simulink model "generic_truck_src"  (Simulink 10.3)
settings: Solver=ode45  StartTime=0.0  StopTime=inf  RelTol=1e-3  EnableMultiTasking=on
libraries: TruckMaker4SL x1, simulink x1
(part 2 of 2)

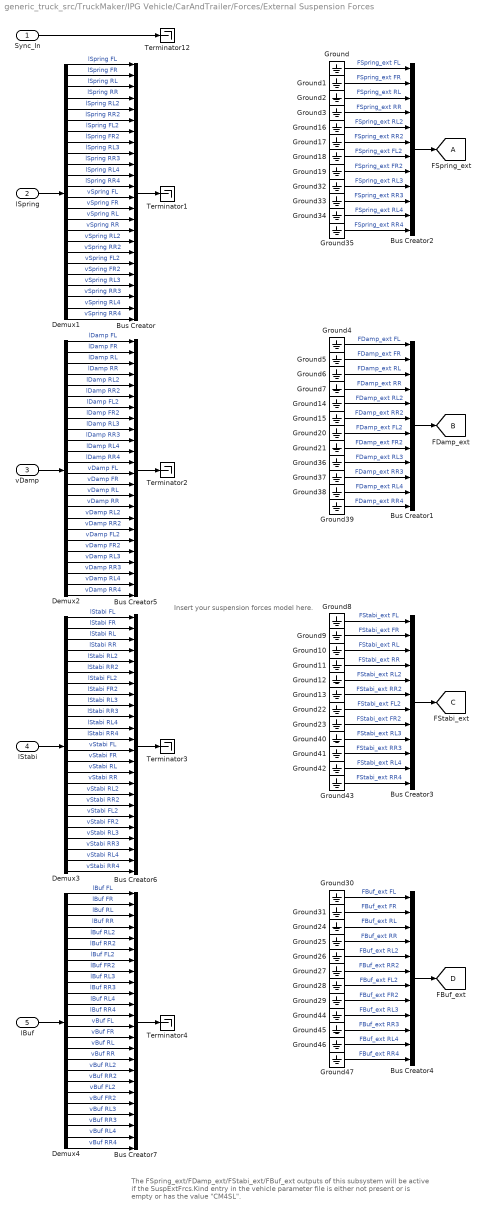
== system generic_truck_src/TruckMaker/IPG Vehicle/CarAndTrailer/Forces/External Suspension Forces ==
  note: The FSpring_ext/FDamp_ext/FStabi_ext/FBuf_ext outputs of this subsystem will be
      | active if the SuspExtFrcs.Kind entry in the vehicle parameter file
      | is either not present or is empty or has the value "CM4SL".
  note: Insert your suspension forces model here.
  Sync_In : Inport
  lSpring : Inport  Port=2
  vDamp : Inport  Port=3
  lStabi : Inport  Port=4
  lBuf : Inport  Port=5
  Bus Creator{,5..7} (4 alike) : BusCreator  Inputs=24
  Bus Creator{1..4} (4 alike) : BusCreator  Inputs=12
  Demux{1..4} (4 alike) : Demux  Outputs=24
      settings: DisplayOption=none
  Ground{,1..47} (48 alike) : Ground
  Terminator{1..4,12} (5 alike) : Terminator
  tag scope: A=global, B=global, C=global, D=global
  wires:
  Ground46/1 -> Bus Creator4/11  "FBuf_ext RL4"
  Ground47/1 -> Bus Creator4/12  "FBuf_ext RR4"
  Ground45/1 -> Bus Creator4/10  "FBuf_ext RR3"
  Ground44/1 -> Bus Creator4/9  "FBuf_ext RL3"
  Ground42/1 -> Bus Creator3/11  "FStabi_ext RL4"
  Ground43/1 -> Bus Creator3/12  "FStabi_ext RR4"
  Ground41/1 -> Bus Creator3/10  "FStabi_ext RR3"
  Ground40/1 -> Bus Creator3/9  "FStabi_ext RL3"
  Ground38/1 -> Bus Creator1/11  "FDamp_ext RL4"
  Ground39/1 -> Bus Creator1/12  "FDamp_ext RR4"
  Ground37/1 -> Bus Creator1/10  "FDamp_ext RR3"
  Ground36/1 -> Bus Creator1/9  "FDamp_ext RL3"
  Ground35/1 -> Bus Creator2/12  "FSpring_ext RR4"
  Ground34/1 -> Bus Creator2/11  "FSpring_ext RL4"
  Ground33/1 -> Bus Creator2/10  "FSpring_ext RR3"
  Ground32/1 -> Bus Creator2/9  "FSpring_ext RL3"
  Demux4/24 -> Bus Creator7/24  "vBuf RR4"
  Demux4/23 -> Bus Creator7/23  "vBuf RL4"
  Demux4/22 -> Bus Creator7/22  "vBuf RR3"
  Demux4/21 -> Bus Creator7/21  "vBuf RL3"
  Demux4/20 -> Bus Creator7/20  "vBuf FR2"
  Demux4/19 -> Bus Creator7/19  "vBuf FL2"
  Demux4/18 -> Bus Creator7/18  "vBuf RR2"
  Demux4/17 -> Bus Creator7/17  "vBuf RL2"
  Demux3/24 -> Bus Creator6/24  "vStabi RR4"
  Demux3/23 -> Bus Creator6/23  "vStabi RL4"
  Demux3/22 -> Bus Creator6/22  "vStabi RR3"
  Demux3/21 -> Bus Creator6/21  "vStabi RL3"
  Demux3/20 -> Bus Creator6/20  "vStabi FR2"
  Demux3/19 -> Bus Creator6/19  "vStabi FL2"
  Demux3/18 -> Bus Creator6/18  "vStabi RR2"
  Demux3/17 -> Bus Creator6/17  "vStabi RL2"
  Demux2/24 -> Bus Creator5/24  "vDamp RR4"
  Demux2/23 -> Bus Creator5/23  "vDamp RL4"
  Demux2/22 -> Bus Creator5/22  "vDamp RR3"
  Demux2/21 -> Bus Creator5/21  "vDamp RL3"
  Demux2/20 -> Bus Creator5/20  "vDamp FR2"
  Demux2/19 -> Bus Creator5/19  "vDamp FL2"
  Demux2/18 -> Bus Creator5/18  "vDamp RR2"
  Demux2/17 -> Bus Creator5/17  "vDamp RL2"
  Demux1/24 -> Bus Creator/24  "vSpring RR4"
  Demux1/23 -> Bus Creator/23  "vSpring RL4"
  Demux1/22 -> Bus Creator/22  "vSpring RR3"
  Demux1/21 -> Bus Creator/21  "vSpring RL3"
  Demux1/20 -> Bus Creator/20  "vSpring FR2"
  Demux1/19 -> Bus Creator/19  "vSpring FL2"
  Demux1/18 -> Bus Creator/18  "vSpring RR2"
  Demux1/17 -> Bus Creator/17  "vSpring RL2"
  Demux3/10 -> Bus Creator6/10  "lStabi RR3"
  Demux4/16 -> Bus Creator7/16  "vBuf RR"
  Demux4/15 -> Bus Creator7/15  "vBuf RL"
  Demux4/14 -> Bus Creator7/14  "vBuf FR"
  Demux4/13 -> Bus Creator7/13  "vBuf FL"
  Demux4/12 -> Bus Creator7/12  "lBuf RR4"
  Demux4/11 -> Bus Creator7/11  "lBuf RL4"
  Demux4/10 -> Bus Creator7/10  "lBuf RR3"
  Demux4/9 -> Bus Creator7/9  "lBuf RL3"
  Demux3/16 -> Bus Creator6/16  "vStabi RR"
  Demux3/15 -> Bus Creator6/15  "vStabi RL"
  Demux3/14 -> Bus Creator6/14  "vStabi FR"
  Demux3/13 -> Bus Creator6/13  "vStabi FL"
  Demux3/12 -> Bus Creator6/12  "lStabi RR4"
  Demux3/11 -> Bus Creator6/11  "lStabi RL4"
  Demux3/9 -> Bus Creator6/9  "lStabi RL3"
  Bus Creator6/1 -> Terminator3/1
  Bus Creator7/1 -> Terminator4/1
  Bus Creator5/1 -> Terminator2/1
  Bus Creator/1 -> Terminator1/1
  Demux2/16 -> Bus Creator5/16  "vDamp RR"
  Demux2/15 -> Bus Creator5/15  "vDamp RL"
  Demux2/14 -> Bus Creator5/14  "vDamp FR"
  Demux2/13 -> Bus Creator5/13  "vDamp FL"
  Demux2/12 -> Bus Creator5/12  "lDamp RR4"
  Demux2/11 -> Bus Creator5/11  "lDamp RL4"
  Demux2/10 -> Bus Creator5/10  "lDamp RR3"
  Demux2/9 -> Bus Creator5/9  "lDamp RL3"
  Demux1/16 -> Bus Creator/16  "vSpring RR"
  Demux1/15 -> Bus Creator/15  "vSpring RL"
  Demux1/14 -> Bus Creator/14  "vSpring FR"
  Demux1/13 -> Bus Creator/13  "vSpring FL"
  Demux1/12 -> Bus Creator/12  "lSpring RR4"
  Demux1/11 -> Bus Creator/11  "lSpring RL4"
  Demux1/10 -> Bus Creator/10  "lSpring RR3"
  Demux1/9 -> Bus Creator/9  "lSpring RL3"
  Demux3/7 -> Bus Creator6/7  "lStabi FL2"
  Demux3/8 -> Bus Creator6/8  "lStabi FR2"
  Ground22/1 -> Bus Creator3/7  "FStabi_ext FL2"
  Ground23/1 -> Bus Creator3/8  "FStabi_ext FR2"
  Demux2/7 -> Bus Creator5/7  "lDamp FL2"
  Demux2/8 -> Bus Creator5/8  "lDamp FR2"
  Ground20/1 -> Bus Creator1/7  "FDamp_ext FL2"
  Ground21/1 -> Bus Creator1/8  "FDamp_ext FR2"
  Ground18/1 -> Bus Creator2/7  "FSpring_ext FL2"
  Ground19/1 -> Bus Creator2/8  "FSpring_ext FR2"
  Demux1/7 -> Bus Creator/7  "lSpring FL2"
  Demux1/8 -> Bus Creator/8  "lSpring FR2"
  Sync_In/1 -> Terminator12/1
  lSpring/1 -> Demux1/1
  vDamp/1 -> Demux2/1
  lStabi/1 -> Demux3/1
  Demux3/1 -> Bus Creator6/1  "lStabi FL"
  Demux3/2 -> Bus Creator6/2  "lStabi FR"
  Demux3/3 -> Bus Creator6/3  "lStabi RL"
  Demux3/4 -> Bus Creator6/4  "lStabi RR"
  Demux1/1 -> Bus Creator/1  "lSpring FL"
  Demux1/2 -> Bus Creator/2  "lSpring FR"
  Demux1/3 -> Bus Creator/3  "lSpring RL"
  Demux1/4 -> Bus Creator/4  "lSpring RR"
  Demux2/1 -> Bus Creator5/1  "lDamp FL"
  Demux2/2 -> Bus Creator5/2  "lDamp FR"
  Demux2/3 -> Bus Creator5/3  "lDamp RL"
  Demux2/4 -> Bus Creator5/4  "lDamp RR"
  Bus Creator2/1 -> [A]
  Ground/1 -> Bus Creator2/1  "FSpring_ext FL"
  Ground1/1 -> Bus Creator2/2  "FSpring_ext FR"
  Ground2/1 -> Bus Creator2/3  "FSpring_ext RL"
  Ground3/1 -> Bus Creator2/4  "FSpring_ext RR"
  Ground4/1 -> Bus Creator1/1  "FDamp_ext FL"
  Ground5/1 -> Bus Creator1/2  "FDamp_ext FR"
  Ground6/1 -> Bus Creator1/3  "FDamp_ext RL"
  Ground7/1 -> Bus Creator1/4  "FDamp_ext RR"
  Bus Creator1/1 -> [B]
  Ground8/1 -> Bus Creator3/1  "FStabi_ext FL"
  Ground9/1 -> Bus Creator3/2  "FStabi_ext FR"
  Ground10/1 -> Bus Creator3/3  "FStabi_ext RL"
  Ground11/1 -> Bus Creator3/4  "FStabi_ext RR"
  Bus Creator3/1 -> [C]
  Demux3/5 -> Bus Creator6/5  "lStabi RL2"
  Demux3/6 -> Bus Creator6/6  "lStabi RR2"
  Ground12/1 -> Bus Creator3/5  "FStabi_ext RL2"
  Ground13/1 -> Bus Creator3/6  "FStabi_ext RR2"
  Demux2/5 -> Bus Creator5/5  "lDamp RL2"
  Demux2/6 -> Bus Creator5/6  "lDamp RR2"
  Ground14/1 -> Bus Creator1/5  "FDamp_ext RL2"
  Ground15/1 -> Bus Creator1/6  "FDamp_ext RR2"
  Demux1/5 -> Bus Creator/5  "lSpring RL2"
  Demux1/6 -> Bus Creator/6  "lSpring RR2"
  Ground16/1 -> Bus Creator2/5  "FSpring_ext RL2"
  Ground17/1 -> Bus Creator2/6  "FSpring_ext RR2"
  Demux4/7 -> Bus Creator7/7  "lBuf FL2"
  Demux4/8 -> Bus Creator7/8  "lBuf FR2"
  Ground28/1 -> Bus Creator4/7  "FBuf_ext FL2"
  Ground29/1 -> Bus Creator4/8  "FBuf_ext FR2"
  lBuf/1 -> Demux4/1
  Demux4/1 -> Bus Creator7/1  "lBuf FL"
  Demux4/2 -> Bus Creator7/2  "lBuf FR"
  Demux4/3 -> Bus Creator7/3  "lBuf RL"
  Demux4/4 -> Bus Creator7/4  "lBuf RR"
  Ground30/1 -> Bus Creator4/1  "FBuf_ext FL"
  Ground31/1 -> Bus Creator4/2  "FBuf_ext FR"
  Ground24/1 -> Bus Creator4/3  "FBuf_ext RL"
  Ground25/1 -> Bus Creator4/4  "FBuf_ext RR"
  Bus Creator4/1 -> [D]
  Demux4/5 -> Bus Creator7/5  "lBuf RL2"
  Demux4/6 -> Bus Creator7/6  "lBuf RR2"
  Ground26/1 -> Bus Creator4/5  "FBuf_ext RL2"
  Ground27/1 -> Bus Creator4/6  "FBuf_ext RR2"

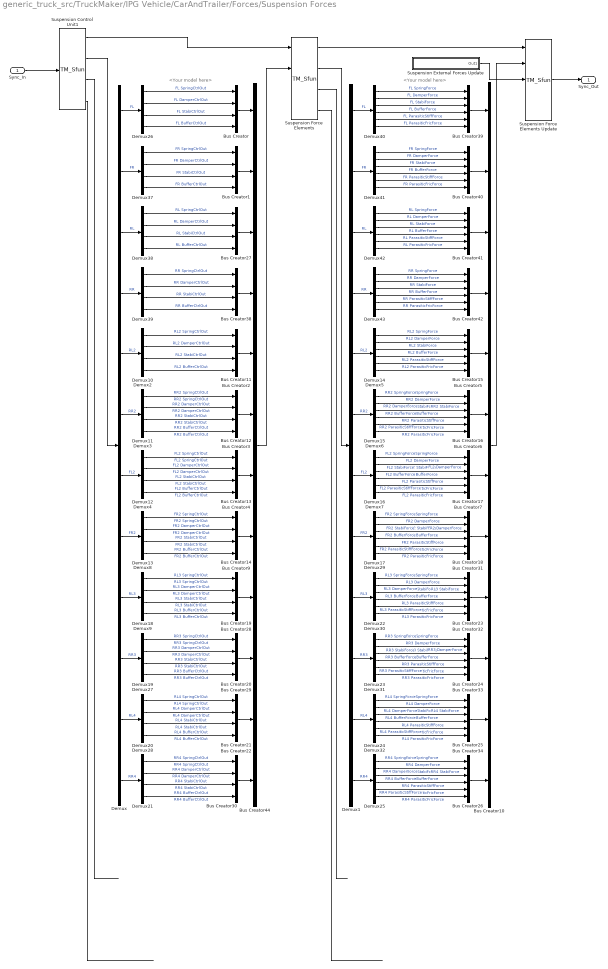
== system generic_truck_src/TruckMaker/IPG Vehicle/CarAndTrailer/Forces/Suspension Forces ==
  note: <Your model here>
  note: <Your model here>
  Sync_In : Inport
  Bus Creator{,1..4,9,11..14,19..22,27..30,38} (19 alike) : BusCreator  Inputs=4
  Bus Creator10 : BusCreator  Inputs=12
  Bus Creator{5..7,15..18,23..26,31..34,39..42} (19 alike) : BusCreator  Inputs=6
  Bus Creator44 : BusCreator  Inputs=12
  Demux : Demux  Outputs=12
  Demux1 : Demux  Outputs=12
  Demux{2..4,8..13,18..21,26..28,37..39} (19 alike) : Demux
  Demux{5..7,14..17,22..25,29..32,40..43} (19 alike) : Demux  Outputs=6
  Suspension Control Unit1 : S-Function  FunctionName=TM_Sfun  Parameters='ForcesSuspControl'  SFunctionDeploymentMode=off  EnableBusSupport=off
  Suspension External Forces Update : Subsystem
  Suspension Force Elements : S-Function  FunctionName=TM_Sfun  Parameters='ForcesSusp'  SFunctionDeploymentMode=off  EnableBusSupport=off
  Suspension Force Elements Update : S-Function  FunctionName=TM_Sfun  Parameters='ForcesSuspUpd'  SFunctionDeploymentMode=off  EnableBusSupport=off
  Sync_Out : Outport  VectorParamsAs1DForOutWhenUnconnected=off
  wires:
  Bus Creator26/1 -> ?
  Bus Creator25/1 -> ?
  Bus Creator24/1 -> ?
  Bus Creator23/1 -> ?
  ? -> Demux25/1  "RR4"
  ? -> Demux24/1  "RL4"
  ? -> Demux23/1  "RR3"
  ? -> Demux22/1  "RL3"
  Demux24/6 -> Bus Creator25/6  "RL4 ParasiticFricForce"
  Demux24/5 -> Bus Creator25/5  "RL4 ParasiticStiffForce"
  Demux24/4 -> Bus Creator25/4  "RL4 BufferForce"
  Demux24/3 -> Bus Creator25/3  "RL4 StabiForce"
  Demux24/2 -> Bus Creator25/2  "RL4 DamperForce"
  Demux25/6 -> Bus Creator26/6  "RR4 ParasiticFricForce"
  Demux25/5 -> Bus Creator26/5  "RR4 ParasiticStiffForce"
  Demux25/4 -> Bus Creator26/4  "RR4 BufferForce"
  Demux25/3 -> Bus Creator26/3  "RR4 StabiForce"
  Demux25/2 -> Bus Creator26/2  "RR4 DamperForce"
  Demux25/1 -> Bus Creator26/1  "RR4 SpringForce"
  Demux24/1 -> Bus Creator25/1  "RL4 SpringForce"
  Demux22/1 -> Bus Creator23/1  "RL3 SpringForce"
  Demux23/1 -> Bus Creator24/1  "RR3 SpringForce"
  Demux23/2 -> Bus Creator24/2  "RR3 DamperForce"
  Demux23/3 -> Bus Creator24/3  "RR3 StabiForce"
  Demux23/4 -> Bus Creator24/4  "RR3 BufferForce"
  Demux23/5 -> Bus Creator24/5  "RR3 ParasiticStiffForce"
  Demux23/6 -> Bus Creator24/6  "RR3 ParasiticFricForce"
  Demux22/2 -> Bus Creator23/2  "RL3 DamperForce"
  Demux22/3 -> Bus Creator23/3  "RL3 StabiForce"
  Demux22/4 -> Bus Creator23/4  "RL3 BufferForce"
  Demux22/5 -> Bus Creator23/5  "RL3 ParasiticStiffForce"
  Demux22/6 -> Bus Creator23/6  "RL3 ParasiticFricForce"
  ? -> Demux21/1  "RR4"
  ? -> Demux20/1  "RL4"
  Bus Creator21/1 -> ?
  Demux20/4 -> Bus Creator21/4  "RL4 BufferCtrlOut"
  Demux20/3 -> Bus Creator21/3  "RL4 StabiCtrlOut"
  Demux20/2 -> Bus Creator21/2  "RL4 DamperCtrlOut"
  Demux21/4 -> Bus Creator22/4  "RR4 BufferCtrlOut"
  Demux21/3 -> Bus Creator22/3  "RR4 StabiCtrlOut"
  Demux21/2 -> Bus Creator22/2  "RR4 DamperCtrlOut"
  Demux21/1 -> Bus Creator22/1  "RR4 SpringCtrlOut"
  Demux20/1 -> Bus Creator21/1  "RL4 SpringCtrlOut"
  Bus Creator22/1 -> ?
  ? -> Demux18/1  "RL3"
  Bus Creator20/1 -> ?
  ? -> Demux19/1  "RR3"
  Demux18/1 -> Bus Creator19/1  "RL3 SpringCtrlOut"
  Demux19/1 -> Bus Creator20/1  "RR3 SpringCtrlOut"
  Demux19/2 -> Bus Creator20/2  "RR3 DamperCtrlOut"
  Demux19/3 -> Bus Creator20/3  "RR3 StabiCtrlOut"
  Demux19/4 -> Bus Creator20/4  "RR3 BufferCtrlOut"
  Demux18/2 -> Bus Creator19/2  "RL3 DamperCtrlOut"
  Demux18/3 -> Bus Creator19/3  "RL3 StabiCtrlOut"
  Demux18/4 -> Bus Creator19/4  "RL3 BufferCtrlOut"
  Bus Creator19/1 -> ?
  ? -> Demux17/1  "FR2"
  ? -> Demux16/1  "FL2"
  ? -> Demux15/1  "RR2"
  Demux15/6 -> Bus Creator16/6  "RR2 ParasiticFricForce"
  Demux15/5 -> Bus Creator16/5  "RR2 ParasiticStiffForce"
  Demux15/4 -> Bus Creator16/4  "RR2 BufferForce"
  Demux15/3 -> Bus Creator16/3  "RR2 StabiForce"
  Demux15/2 -> Bus Creator16/2  "RR2 DamperForce"
  Demux15/1 -> Bus Creator16/1  "RR2 SpringForce"
  Demux16/3 -> Bus Creator17/3  "FL2 StabiForce"
  Demux16/6 -> Bus Creator17/6  "FL2 ParasiticFricForce"
  Demux16/5 -> Bus Creator17/5  "FL2 ParasiticStiffForce"
  Demux16/4 -> Bus Creator17/4  "FL2 BufferForce"
  Demux16/2 -> Bus Creator17/2  "FL2 DamperForce"
  Demux16/1 -> Bus Creator17/1  "FL2 SpringForce"
  Demux17/6 -> Bus Creator18/6  "FR2 ParasiticFricForce"
  Demux17/5 -> Bus Creator18/5  "FR2 ParasiticStiffForce"
  Demux17/4 -> Bus Creator18/4  "FR2 BufferForce"
  Demux17/3 -> Bus Creator18/3  "FR2 StabiForce"
  Demux17/2 -> Bus Creator18/2  "FR2 DamperForce"
  Demux17/1 -> Bus Creator18/1  "FR2 SpringForce"
  Bus Creator18/1 -> ?
  Bus Creator17/1 -> ?
  Bus Creator16/1 -> ?
  Demux11/4 -> Bus Creator12/4  "RR2 BufferCtrlOut"
  Demux11/3 -> Bus Creator12/3  "RR2 StabiCtrlOut"
  Demux11/2 -> Bus Creator12/2  "RR2 DamperCtrlOut"
  Demux11/1 -> Bus Creator12/1  "RR2 SpringCtrlOut"
  Demux12/3 -> Bus Creator13/3  "FL2 StabiCtrlOut"
  Demux12/4 -> Bus Creator13/4  "FL2 BufferCtrlOut"
  Demux12/2 -> Bus Creator13/2  "FL2 DamperCtrlOut"
  Demux12/1 -> Bus Creator13/1  "FL2 SpringCtrlOut"
  Demux13/4 -> Bus Creator14/4  "FR2 BufferCtrlOut"
  Demux13/3 -> Bus Creator14/3  "FR2 StabiCtrlOut"
  Demux13/2 -> Bus Creator14/2  "FR2 DamperCtrlOut"
  Demux13/1 -> Bus Creator14/1  "FR2 SpringCtrlOut"
  ? -> Demux13/1  "FR2"
  Bus Creator14/1 -> ?
  ? -> Demux12/1  "FL2"
  Bus Creator13/1 -> ?
  ? -> Demux11/1  "RR2"
  Bus Creator12/1 -> ?
  Demux7/5 -> Bus Creator7/5  "FR2 ParasiticStiffForce"
  Bus Creator10/1 -> Suspension Force Elements Update/2
  Demux29/1 -> Bus Creator31/1  "RL3 SpringForce"
  Demux37/2 -> Bus Creator1/2  "FR DamperCtrlOut"
  Demux32/1 -> Bus Creator34/1  "RR4 SpringForce"
  Demux37/4 -> Bus Creator1/4  "FR BufferCtrlOut"
  Demux32/2 -> Bus Creator34/2  "RR4 DamperForce"
  Demux2/3 -> Bus Creator2/3  "RR2 StabiCtrlOut"
  Suspension Force Elements/2 -> Demux1/1
  Demux10/1 -> Bus Creator11/1  "RL2 SpringCtrlOut"
  Demux6/4 -> Bus Creator6/4  "FL2 BufferForce"
  Demux14/1 -> Bus Creator15/1  "RL2 SpringForce"
  Suspension External Forces Update/1(Out1) -> Suspension Force Elements Update/3
  Demux30/4 -> Bus Creator32/4  "RR3 BufferForce"
  Demux8/3 -> Bus Creator9/3  "RL3 StabiCtrlOut"
  Demux1/7 -> Demux6/1  "FL2"
  Demux30/3 -> Bus Creator32/3  "RR3 StabiForce"
  Demux8/2 -> Bus Creator9/2  "RL3 DamperCtrlOut"
  Demux30/1 -> Bus Creator32/1  "RR3 SpringForce"
  Demux37/1 -> Bus Creator1/1  "FR SpringCtrlOut"
  Suspension Control Unit1/3 -> ?
  Demux41/6 -> Bus Creator40/6  "FR ParasiticFricForce"
  Demux40/3 -> Bus Creator39/3  "FL StabiForce"
  Demux41/4 -> Bus Creator40/4  "FR BufferForce"
  Demux4/2 -> Bus Creator4/2  "FR2 DamperCtrlOut"
  Demux6/1 -> Bus Creator6/1  "FL2 SpringForce"
  Demux31/4 -> Bus Creator33/4  "RL4 BufferForce"
  Demux1/11 -> Demux31/1  "RL4"
  Demux6/5 -> Bus Creator6/5  "FL2 ParasiticStiffForce"
  Bus Creator3/1 -> Bus Creator44/7
  Demux9/4 -> Bus Creator28/4  "RR3 BufferCtrlOut"
  Demux30/2 -> Bus Creator32/2  "RR3 DamperForce"
  Bus Creator5/1 -> Bus Creator10/6
  Demux9/3 -> Bus Creator28/3  "RR3 StabiCtrlOut"
  Bus Creator4/1 -> Bus Creator44/8
  Demux8/1 -> Bus Creator9/1  "RL3 SpringCtrlOut"
  Demux7/1 -> Bus Creator7/1  "FR2 SpringForce"
  Demux28/1 -> Bus Creator30/1  "RR4 SpringCtrlOut"
  Demux42/5 -> Bus Creator41/5  "RL ParasiticStiffForce"
  Demux43/5 -> Bus Creator42/5  "RR ParasiticStiffForce"
  Demux32/5 -> Bus Creator34/5  "RR4 ParasiticStiffForce"
  Bus Creator39/1 -> Bus Creator10/1
  Demux/6 -> Demux2/1  "RR2"
  Demux37/3 -> Bus Creator1/3  "FR StabiCtrlOut"
  Demux31/1 -> Bus Creator33/1  "RL4 SpringForce"
  Demux42/6 -> Bus Creator41/6  "RL ParasiticFricForce"
  Demux43/6 -> Bus Creator42/6  "RR ParasiticFricForce"
  Demux6/3 -> Bus Creator6/3  "FL2 StabiForce"
  Bus Creator31/1 -> Bus Creator10/9
  Demux38/4 -> Bus Creator27/4  "RL BufferCtrlOut"
  Bus Creator1/1 -> Bus Creator44/2
  Suspension Force Elements/4 -> ?
  Demux5/2 -> Bus Creator5/2  "RR2 DamperForce"
  Suspension Force Elements Update/1 -> Sync_Out/1
  Demux31/6 -> Bus Creator33/6  "RL4 ParasiticFricForce"
  Bus Creator32/1 -> Bus Creator10/10
  Demux3/4 -> Bus Creator3/4  "FL2 BufferCtrlOut"
  Demux1/4 -> Demux43/1  "RR"
  Demux39/3 -> Bus Creator38/3  "RR StabiCtrlOut"
  Demux1/8 -> Demux7/1  "FR2"
  Bus Creator/1 -> Bus Creator44/1
  Demux3/1 -> Bus Creator3/1  "FL2 SpringCtrlOut"
  Demux42/3 -> Bus Creator41/3  "RL StabiForce"
  Demux42/1 -> Bus Creator41/1  "RL SpringForce"
  Suspension Force Elements/1 -> Suspension Force Elements Update/1
  Bus Creator11/1 -> Bus Creator44/5
  Demux32/3 -> Bus Creator34/3  "RR4 StabiForce"
  Demux30/5 -> Bus Creator32/5  "RR3 ParasiticStiffForce"
  Demux32/6 -> Bus Creator34/6  "RR4 ParasiticFricForce"
  Demux40/5 -> Bus Creator39/5  "FL ParasiticStiffForce"
  Demux6/2 -> Bus Creator6/2  "FL2 DamperForce"
  Demux14/2 -> Bus Creator15/2  "RL2 DamperForce"
  Demux32/4 -> Bus Creator34/4  "RR4 BufferForce"
  Demux8/4 -> Bus Creator9/4  "RL3 BufferCtrlOut"
  Demux10/3 -> Bus Creator11/3  "RL2 StabiCtrlOut"
  ? -> Suspension Force Elements Update/4
  Bus Creator30/1 -> Bus Creator44/12
  Bus Creator27/1 -> Bus Creator44/3
  Demux41/1 -> Bus Creator40/1  "FR SpringForce"
  Demux3/2 -> Bus Creator3/2  "FL2 DamperCtrlOut"
  Demux38/2 -> Bus Creator27/2  "RL DamperCtrlOut"
  Demux31/5 -> Bus Creator33/5  "RL4 ParasiticStiffForce"
  Demux43/3 -> Bus Creator42/3  "RR StabiForce"
  Demux43/1 -> Bus Creator42/1  "RR SpringForce"
  Demux26/4 -> Bus Creator/4  "FL BufferCtrlOut"
  Demux27/4 -> Bus Creator29/4  "RL4 BufferCtrlOut"
  Demux1/10 -> Demux30/1  "RR3"
  Demux42/2 -> Bus Creator41/2  "RL DamperForce"
  Demux1/9 -> Demux29/1  "RL3"
  Bus Creator44/1 -> Suspension Force Elements/2
  Demux5/3 -> Bus Creator5/3  "RR2 StabiForce"
  Demux40/2 -> Bus Creator39/2  "FL DamperForce"
  Bus Creator2/1 -> Bus Creator44/6
  Demux43/2 -> Bus Creator42/2  "RR DamperForce"
  Demux/1 -> Demux26/1  "FL"
  Suspension Control Unit1/2 -> Demux/1
  Demux41/2 -> Bus Creator40/2  "FR DamperForce"
  Demux1/12 -> Demux32/1  "RR4"
  Demux14/3 -> Bus Creator15/3  "RL2 StabiForce"
  Demux2/4 -> Bus Creator2/4  "RR2 BufferCtrlOut"
  Demux1/1 -> Demux40/1  "FL"
  Demux/12 -> Demux28/1  "RR4"
  Demux5/1 -> Bus Creator5/1  "RR2 SpringForce"
  Demux2/2 -> Bus Creator2/2  "RR2 DamperCtrlOut"
  Demux2/1 -> Bus Creator2/1  "RR2 SpringCtrlOut"
  Demux1/5 -> Demux14/1  "RL2"
  Demux26/3 -> Bus Creator/3  "FL StabiCtrlOut"
  Demux5/4 -> Bus Creator5/4  "RR2 BufferForce"
  Demux14/4 -> Bus Creator15/4  "RL2 BufferForce"
  Demux40/6 -> Bus Creator39/6  "FL ParasiticFricForce"
  Suspension Control Unit1/1 -> Suspension Force Elements/1
  Bus Creator41/1 -> Bus Creator10/3
  Demux6/6 -> Bus Creator6/6  "FL2 ParasiticFricForce"
  Demux26/2 -> Bus Creator/2  "FL DamperCtrlOut"
  Demux7/6 -> Bus Creator7/6  "FR2 ParasiticFricForce"
  ? -> ?  "tWheelCarrier_z FL"
  Demux4/1 -> Bus Creator4/1  "FR2 SpringCtrlOut"
  Bus Creator33/1 -> Bus Creator10/11
  Demux31/2 -> Bus Creator33/2  "RL4 DamperForce"
  Demux30/6 -> Bus Creator32/6  "RR3 ParasiticFricForce"
  Demux5/5 -> Bus Creator5/5  "RR2 ParasiticStiffForce"
  Demux28/3 -> Bus Creator30/3  "RR4 StabiCtrlOut"
  Demux38/1 -> Bus Creator27/1  "RL SpringCtrlOut"
  Bus Creator40/1 -> Bus Creator10/2
  Bus Creator29/1 -> Bus Creator44/11
  Demux/4 -> Demux39/1  "RR"
  Demux/3 -> Demux38/1  "RL"
  Demux38/3 -> Bus Creator27/3  "RL StabiCtrlOut"
  Demux39/1 -> Bus Creator38/1  "RR SpringCtrlOut"
  Demux5/6 -> Bus Creator5/6  "RR2 ParasiticFricForce"
  Demux40/1 -> Bus Creator39/1  "FL SpringForce"
  Demux27/2 -> Bus Creator29/2  "RL4 DamperCtrlOut"
  Demux10/4 -> Bus Creator11/4  "RL2 BufferCtrlOut"
  Demux41/5 -> Bus Creator40/5  "FR ParasiticStiffForce"
  Demux4/4 -> Bus Creator4/4  "FR2 BufferCtrlOut"
  Demux1/2 -> Demux41/1  "FR"
  Demux9/2 -> Bus Creator28/2  "RR3 DamperCtrlOut"
  Demux39/4 -> Bus Creator38/4  "RR BufferCtrlOut"
  Demux7/3 -> Bus Creator7/3  "FR2 StabiForce"
  Bus Creator42/1 -> Bus Creator10/4
  ? -> Suspension Force Elements Update/5
  Bus Creator6/1 -> Bus Creator10/7
  Demux27/1 -> Bus Creator29/1  "RL4 SpringCtrlOut"
  Sync_In/1 -> Suspension Control Unit1/1
  Demux31/3 -> Bus Creator33/3  "RL4 StabiForce"
  Bus Creator28/1 -> Bus Creator44/10
  Demux42/4 -> Bus Creator41/4  "RL BufferForce"
  Demux43/4 -> Bus Creator42/4  "RR BufferForce"
  ? -> Suspension Force Elements/3
  Demux39/2 -> Bus Creator38/2  "RR DamperCtrlOut"
  Demux14/5 -> Bus Creator15/5  "RL2 ParasiticStiffForce"
  Demux14/6 -> Bus Creator15/6  "RL2 ParasiticFricForce"
  Demux29/4 -> Bus Creator31/4  "RL3 BufferForce"
  Demux7/2 -> Bus Creator7/2  "FR2 DamperForce"
  Bus Creator15/1 -> Bus Creator10/5
  Demux/8 -> Demux4/1  "FR2"
  Demux10/2 -> Bus Creator11/2  "RL2 DamperCtrlOut"
  Demux29/6 -> Bus Creator31/6  "RL3 ParasiticFricForce"
  Demux1/6 -> Demux5/1  "RR2"
  Demux7/4 -> Bus Creator7/4  "FR2 BufferForce"
  Demux/11 -> Demux27/1  "RL4"
  Demux1/3 -> Demux42/1  "RL"
  Demux29/2 -> Bus Creator31/2  "RL3 DamperForce"
  Demux29/3 -> Bus Creator31/3  "RL3 StabiForce"
  Suspension Force Elements/3 -> ?
  Demux29/5 -> Bus Creator31/5  "RL3 ParasiticStiffForce"
  Demux26/1 -> Bus Creator/1  "FL SpringCtrlOut"
  Bus Creator38/1 -> Bus Creator44/4
  ? -> Suspension Force Elements/4
  Bus Creator7/1 -> Bus Creator10/8
  Bus Creator9/1 -> Bus Creator44/9
  Demux28/2 -> Bus Creator30/2  "RR4 DamperCtrlOut"
  Demux/9 -> Demux8/1  "RL3"
  Demux/10 -> Demux9/1  "RR3"
  Bus Creator34/1 -> Bus Creator10/12
  Demux4/3 -> Bus Creator4/3  "FR2 StabiCtrlOut"
  Demux3/3 -> Bus Creator3/3  "FL2 StabiCtrlOut"
  Demux9/1 -> Bus Creator28/1  "RR3 SpringCtrlOut"
  Demux/2 -> Demux37/1  "FR"
  Demux/7 -> Demux3/1  "FL2"
  Demux/5 -> Demux10/1  "RL2"
  Suspension Control Unit1/4 -> ?
  Demux27/3 -> Bus Creator29/3  "RL4 StabiCtrlOut"
  Demux28/4 -> Bus Creator30/4  "RR4 BufferCtrlOut"
  Demux40/4 -> Bus Creator39/4  "FL BufferForce"
  Demux41/3 -> Bus Creator40/3  "FR StabiForce"

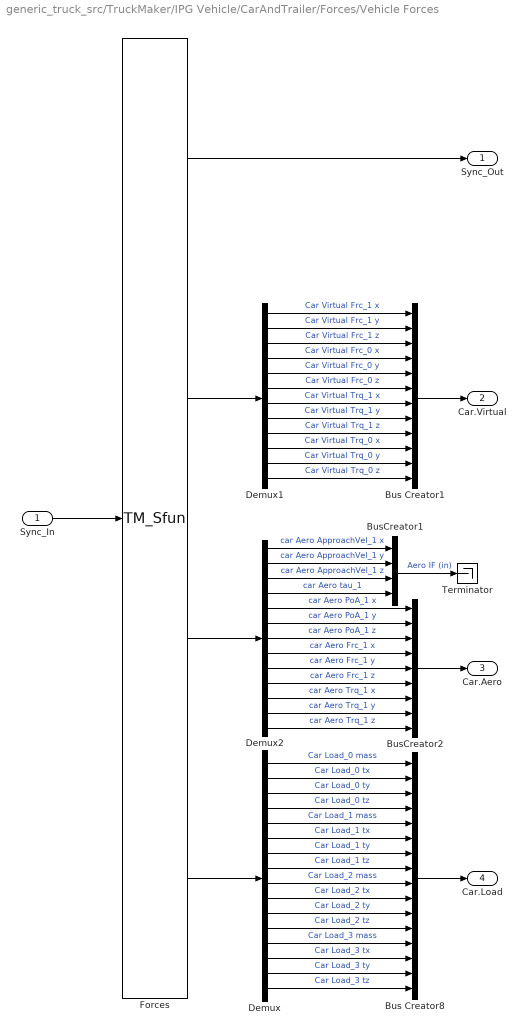
== system generic_truck_src/TruckMaker/IPG Vehicle/CarAndTrailer/Forces/Vehicle Forces ==
  Sync_In : Inport
  Bus Creator1 : BusCreator  Inputs=12
  Bus Creator8 : BusCreator  Inputs=16
  BusCreator1 : BusCreator  Inputs=4
  BusCreator2 : BusCreator  Inputs=9
  Demux : Demux  Outputs=16
      settings: DisplayOption=none
  Demux1 : Demux  Outputs=12
      settings: DisplayOption=none
  Demux2 : Demux  Outputs=13
      settings: DisplayOption=none
  Forces : S-Function  FunctionName=TM_Sfun  Parameters='Forces'  SFunctionDeploymentMode=off  EnableBusSupport=off
  Terminator : Terminator
  Sync_Out : Outport  VectorParamsAs1DForOutWhenUnconnected=off
  Car.Virtual : Outport  Port=2  VectorParamsAs1DForOutWhenUnconnected=off
  Car.Aero : Outport  Port=3  VectorParamsAs1DForOutWhenUnconnected=off
  Car.Load : Outport  Port=4  VectorParamsAs1DForOutWhenUnconnected=off
  wires:
  BusCreator1/1 -> Terminator/1  "Aero IF (in)"
  Demux2/13 -> BusCreator2/9  "car Aero Trq_1 z"
  Demux2/12 -> BusCreator2/8  "car Aero Trq_1 y"
  Demux2/11 -> BusCreator2/7  "car Aero Trq_1 x"
  Demux2/10 -> BusCreator2/6  "car Aero Frc_1 z"
  Demux2/9 -> BusCreator2/5  "car Aero Frc_1 y"
  Demux2/8 -> BusCreator2/4  "car Aero Frc_1 x"
  Demux2/7 -> BusCreator2/3  "car Aero PoA_1 z"
  Demux2/6 -> BusCreator2/2  "car Aero PoA_1 y"
  Demux2/5 -> BusCreator2/1  "car Aero PoA_1 x"
  Demux2/4 -> BusCreator1/4  "car Aero tau_1"
  Demux2/3 -> BusCreator1/3  "car Aero ApproachVel_1 z"
  Demux2/2 -> BusCreator1/2  "car Aero ApproachVel_1 y"
  Demux2/1 -> BusCreator1/1  "car Aero ApproachVel_1 x"
  BusCreator2/1 -> Car.Aero/1
  Demux/16 -> Bus Creator8/16  "Car Load_3 tz"
  Demux/15 -> Bus Creator8/15  "Car Load_3 ty"
  Demux/14 -> Bus Creator8/14  "Car Load_3 tx"
  Demux/13 -> Bus Creator8/13  "Car Load_3 mass"
  Demux1/12 -> Bus Creator1/12  "Car Virtual Trq_0 z"
  Demux1/11 -> Bus Creator1/11  "Car Virtual Trq_0 y"
  Demux1/10 -> Bus Creator1/10  "Car Virtual Trq_0 x"
  Demux1/9 -> Bus Creator1/9  "Car Virtual Trq_1 z"
  Demux1/8 -> Bus Creator1/8  "Car Virtual Trq_1 y"
  Demux1/7 -> Bus Creator1/7  "Car Virtual Trq_1 x"
  Demux1/6 -> Bus Creator1/6  "Car Virtual Frc_0 z"
  Demux1/5 -> Bus Creator1/5  "Car Virtual Frc_0 y"
  Demux1/4 -> Bus Creator1/4  "Car Virtual Frc_0 x"
  Sync_In/1 -> Forces/1
  Forces/1 -> Sync_Out/1
  Demux1/1 -> Bus Creator1/1  "Car Virtual Frc_1 x"
  Demux1/2 -> Bus Creator1/2  "Car Virtual Frc_1 y"
  Demux1/3 -> Bus Creator1/3  "Car Virtual Frc_1 z"
  Forces/3 -> Demux2/1
  Forces/2 -> Demux1/1
  Bus Creator1/1 -> Car.Virtual/1
  Bus Creator8/1 -> Car.Load/1
  Demux/1 -> Bus Creator8/1  "Car Load_0 mass"
  Demux/2 -> Bus Creator8/2  "Car Load_0 tx"
  Demux/3 -> Bus Creator8/3  "Car Load_0 ty"
  Demux/4 -> Bus Creator8/4  "Car Load_0 tz"
  Demux/5 -> Bus Creator8/5  "Car Load_1 mass"
  Demux/6 -> Bus Creator8/6  "Car Load_1 tx"
  Demux/7 -> Bus Creator8/7  "Car Load_1 ty"
  Demux/8 -> Bus Creator8/8  "Car Load_1 tz"
  Demux/9 -> Bus Creator8/9  "Car Load_2 mass"
  Demux/10 -> Bus Creator8/10  "Car Load_2 tx"
  Demux/11 -> Bus Creator8/11  "Car Load_2 ty"
  Demux/12 -> Bus Creator8/12  "Car Load_2 tz"
  Forces/4 -> Demux/1

== system generic_truck_src/TruckMaker/IPG Vehicle/CarAndTrailer/Trailer/CreateBus Car.Hitch.FrcTrq ==
  In1 : Inport
  Bus Creator7 : BusCreator  Inputs=6
  Demux7 : Demux  Outputs=6
      settings: DisplayOption=none
  Out1 : Outport  VectorParamsAs1DForOutWhenUnconnected=off
  wires:
  In1/1 -> Demux7/1
  Bus Creator7/1 -> Out1/1
  Demux7/6 -> Bus Creator7/6  "Car Hitch Trq2Car z"
  Demux7/5 -> Bus Creator7/5  "Car Hitch Trq2Car y"
  Demux7/4 -> Bus Creator7/4  "Car Hitch Trq2Car x"
  Demux7/3 -> Bus Creator7/3  "Car Hitch Frc2Car z"
  Demux7/2 -> Bus Creator7/2  "Car Hitch Frc2Car y"
  Demux7/1 -> Bus Creator7/1  "Car Hitch Frc2Car x"

== system generic_truck_src/TruckMaker/IPG Vehicle/CarAndTrailer/Trailer/CreateBus Vhcl.Motion ==
  In1 : Inport
  BusCreator : BusCreator  Inputs=15
  Demux : Demux  Outputs=15
      settings: DisplayOption=none
  Out1 : Outport  VectorParamsAs1DForOutWhenUnconnected=off
  wires:
  Demux/15 -> BusCreator/15  "Vhcl YawAcc"
  Demux/14 -> BusCreator/14  "Vhcl YawVel"
  Demux/13 -> BusCreator/13  "Vhcl Yaw"
  Demux/12 -> BusCreator/12  "Vhcl PitchAcc"
  Demux/11 -> BusCreator/11  "Vhcl PitchVel"
  Demux/10 -> BusCreator/10  "Vhcl Pitch"
  Demux/9 -> BusCreator/9  "Vhcl RollAcc"
  Demux/8 -> BusCreator/8  "Vhcl RollVel"
  Demux/7 -> BusCreator/7  "Vhcl Roll"
  Demux/6 -> BusCreator/6  "Vhcl Hitch_Pos z"
  Demux/5 -> BusCreator/5  "Vhcl Hitch_Pos y"
  Demux/4 -> BusCreator/4  "Vhcl Hitch_Pos x"
  Demux/3 -> BusCreator/3  "Vhcl sRoad"
  Demux/2 -> BusCreator/2  "Vhcl Distance"
  Demux/1 -> BusCreator/1  "Vhcl v"
  In1/1 -> Demux/1
  BusCreator/1 -> Out1/1

== system generic_truck_src/TruckMaker/IPG Vehicle/CarAndTrailer/Trailer/CreateBus Vhcl.PoI ==
  In1 : Inport
  Bus Creator3 : BusCreator  Inputs=18
  Demux3 : Demux  Outputs=18
      settings: DisplayOption=none
  Out1 : Outport  VectorParamsAs1DForOutWhenUnconnected=off
  wires:
  Demux3/18 -> Bus Creator3/18  "Vhcl PoI_GCS Elev"
  Demux3/17 -> Bus Creator3/17  "Vhcl PoI_GCS Lat"
  Demux3/16 -> Bus Creator3/16  "Vhcl PoI_GCS Long"
  Demux3/15 -> Bus Creator3/15  "Vhcl PoI_Acc_1 z"
  Demux3/14 -> Bus Creator3/14  "Vhcl PoI_Acc_1 y"
  Demux3/13 -> Bus Creator3/13  "Vhcl PoI_Acc_1 x"
  Demux3/12 -> Bus Creator3/12  "Vhcl PoI_Vel_1 z"
  Demux3/11 -> Bus Creator3/11  "Vhcl PoI_Vel_1 y"
  Demux3/10 -> Bus Creator3/10  "Vhcl PoI_Vel_1 x"
  Demux3/9 -> Bus Creator3/9  "Vhcl PoI_Acc z"
  Demux3/8 -> Bus Creator3/8  "Vhcl PoI_Acc y"
  Demux3/7 -> Bus Creator3/7  "Vhcl PoI_Acc x"
  Demux3/6 -> Bus Creator3/6  "Vhcl PoI_Vel z"
  Demux3/5 -> Bus Creator3/5  "Vhcl PoI_Vel y"
  Demux3/4 -> Bus Creator3/4  "Vhcl PoI_Vel x"
  Demux3/3 -> Bus Creator3/3  "Vhcl PoI_Pos z"
  Demux3/2 -> Bus Creator3/2  "Vhcl PoI_Pos y"
  In1/1 -> Demux3/1
  Bus Creator3/1 -> Out1/1
  Demux3/1 -> Bus Creator3/1  "Vhcl PoI_Pos x"

== system generic_truck_src/TruckMaker/IPG Vehicle/CarAndTrailer/Trailer/CreateBus Vhcl.Steering ==
  In1 : Inport
  Bus Creator3 : BusCreator  Inputs=4
  Demux : Demux
      settings: DisplayOption=none
  Out1 : Outport  VectorParamsAs1DForOutWhenUnconnected=off
  wires:
  Bus Creator3/1 -> Out1/1
  Demux/1 -> Bus Creator3/1  "Vhcl Steering Ang"
  Demux/3 -> Bus Creator3/3  "Vhcl Steering AngAcc"
  Demux/2 -> Bus Creator3/2  "Vhcl Steering AngVel"
  Demux/4 -> Bus Creator3/4  "Vhcl Steering Trq"
  In1/1 -> Demux/1

== system generic_truck_src/TruckMaker/IPG Vehicle/CarAndTrailer/Trailer/CreateBus Vhcl.Wheel.FL ==
  In1 : Inport
  Bus Creator3 : BusCreator  Inputs=14
  Demux3 : Demux  Outputs=14
      settings: DisplayOption=none
  Out1 : Outport  VectorParamsAs1DForOutWhenUnconnected=off
  wires:
  Demux3/14 -> Bus Creator3/14  "Vhcl Wheel FL Trq_WhlBearing"
  Demux3/13 -> Bus Creator3/13  "Vhcl Wheel FL Trq_T2W"
  Demux3/12 -> Bus Creator3/12  "Vhcl Wheel FL SideSlip"
  Demux3/11 -> Bus Creator3/11  "Vhcl Wheel FL LongSlip"
  Demux3/10 -> Bus Creator3/10  "Vhcl Wheel FL vBelt"
  Demux3/9 -> Bus Creator3/9  "Vhcl Wheel FL Fz"
  Demux3/8 -> Bus Creator3/8  "Vhcl Wheel FL Fy"
  Demux3/7 -> Bus Creator3/7  "Vhcl Wheel FL Fx"
  Demux3/6 -> Bus Creator3/6  "Vhcl Wheel FL r_zxy z"
  Demux3/5 -> Bus Creator3/5  "Vhcl Wheel FL r_zxy y"
  Demux3/4 -> Bus Creator3/4  "Vhcl Wheel FL r_zxy x"
  Demux3/3 -> Bus Creator3/3  "Vhcl Wheel FL t z"
  Demux3/2 -> Bus Creator3/2  "Vhcl Wheel FL t y"
  In1/1 -> Demux3/1
  Bus Creator3/1 -> Out1/1
  Demux3/1 -> Bus Creator3/1  "Vhcl Wheel FL t x"

== system generic_truck_src/TruckMaker/IPG Vehicle/CarAndTrailer/Trailer/CreateBus Vhcl.Wheel.FL2 ==
  In1 : Inport
  Bus Creator3 : BusCreator  Inputs=14
  Demux3 : Demux  Outputs=14
      settings: DisplayOption=none
  Out1 : Outport  VectorParamsAs1DForOutWhenUnconnected=off
  wires:
  Demux3/14 -> Bus Creator3/14  "Vhcl Wheel FL2 Trq_WhlBearing"
  Demux3/13 -> Bus Creator3/13  "Vhcl Wheel FL2 Trq_T2W"
  Demux3/12 -> Bus Creator3/12  "Vhcl Wheel FL2 SideSlip"
  Demux3/11 -> Bus Creator3/11  "Vhcl Wheel FL2 LongSlip"
  Demux3/10 -> Bus Creator3/10  "Vhcl Wheel FL2 vBelt"
  Demux3/9 -> Bus Creator3/9  "Vhcl Wheel FL2 Fz"
  Demux3/8 -> Bus Creator3/8  "Vhcl Wheel FL2 Fy"
  Demux3/7 -> Bus Creator3/7  "Vhcl Wheel FL2 Fx"
  Demux3/6 -> Bus Creator3/6  "Vhcl Wheel FL2 r_zxy z"
  Demux3/5 -> Bus Creator3/5  "Vhcl Wheel FL2 r_zxy y"
  Demux3/4 -> Bus Creator3/4  "Vhcl Wheel FL2 r_zxy x"
  Demux3/3 -> Bus Creator3/3  "Vhcl Wheel FL2 t z"
  Demux3/2 -> Bus Creator3/2  "Vhcl Wheel FL2 t y"
  In1/1 -> Demux3/1
  Bus Creator3/1 -> Out1/1
  Demux3/1 -> Bus Creator3/1  "Vhcl Wheel FL2 t x"

== system generic_truck_src/TruckMaker/IPG Vehicle/CarAndTrailer/Trailer/CreateBus Vhcl.Wheel.FR ==
  In1 : Inport
  Bus Creator3 : BusCreator  Inputs=14
  Demux3 : Demux  Outputs=14
      settings: DisplayOption=none
  Out1 : Outport  VectorParamsAs1DForOutWhenUnconnected=off
  wires:
  Demux3/14 -> Bus Creator3/14  "Vhcl Wheel FR Trq_WhlBearing"
  Demux3/13 -> Bus Creator3/13  "Vhcl Wheel FR Trq_T2W"
  Demux3/12 -> Bus Creator3/12  "Vhcl Wheel FR SideSlip"
  Demux3/11 -> Bus Creator3/11  "Vhcl Wheel FR LongSlip"
  Demux3/10 -> Bus Creator3/10  "Vhcl Wheel FR vBelt"
  Demux3/9 -> Bus Creator3/9  "Vhcl Wheel FR Fz"
  Demux3/8 -> Bus Creator3/8  "Vhcl Wheel FR Fy"
  Demux3/7 -> Bus Creator3/7  "Vhcl Wheel FR Fx"
  Demux3/6 -> Bus Creator3/6  "Vhcl Wheel FR r_zxy z"
  Demux3/5 -> Bus Creator3/5  "Vhcl Wheel FR r_zxy y"
  Demux3/4 -> Bus Creator3/4  "Vhcl Wheel FR r_zxy x"
  Demux3/3 -> Bus Creator3/3  "Vhcl Wheel FR t z"
  Demux3/2 -> Bus Creator3/2  "Vhcl Wheel FR t y"
  In1/1 -> Demux3/1
  Bus Creator3/1 -> Out1/1
  Demux3/1 -> Bus Creator3/1  "Vhcl Wheel FR t x"

== system generic_truck_src/TruckMaker/IPG Vehicle/CarAndTrailer/Trailer/CreateBus Vhcl.Wheel.FR2 ==
  In1 : Inport
  Bus Creator3 : BusCreator  Inputs=14
  Demux3 : Demux  Outputs=14
      settings: DisplayOption=none
  Out1 : Outport  VectorParamsAs1DForOutWhenUnconnected=off
  wires:
  Demux3/14 -> Bus Creator3/14  "Vhcl Wheel FR2 Trq_WhlBearing"
  Demux3/13 -> Bus Creator3/13  "Vhcl Wheel FR2 Trq_T2W"
  Demux3/12 -> Bus Creator3/12  "Vhcl Wheel FR2 SideSlip"
  Demux3/11 -> Bus Creator3/11  "Vhcl Wheel FR2 LongSlip"
  Demux3/10 -> Bus Creator3/10  "Vhcl Wheel FR2 vBelt"
  Demux3/9 -> Bus Creator3/9  "Vhcl Wheel FR2 Fz"
  Demux3/8 -> Bus Creator3/8  "Vhcl Wheel FR2 Fy"
  Demux3/7 -> Bus Creator3/7  "Vhcl Wheel FR2 Fx"
  Demux3/6 -> Bus Creator3/6  "Vhcl Wheel FR2 r_zxy z"
  Demux3/5 -> Bus Creator3/5  "Vhcl Wheel FR2 r_zxy y"
  Demux3/4 -> Bus Creator3/4  "Vhcl Wheel FR2 r_zxy x"
  Demux3/3 -> Bus Creator3/3  "Vhcl Wheel FR2 t z"
  Demux3/2 -> Bus Creator3/2  "Vhcl Wheel FR2 t y"
  In1/1 -> Demux3/1
  Bus Creator3/1 -> Out1/1
  Demux3/1 -> Bus Creator3/1  "Vhcl Wheel FR2 t x"

== system generic_truck_src/TruckMaker/IPG Vehicle/CarAndTrailer/Trailer/CreateBus Vhcl.Wheel.RL ==
  In1 : Inport
  Bus Creator3 : BusCreator  Inputs=14
  Demux3 : Demux  Outputs=14
      settings: DisplayOption=none
  Out1 : Outport  VectorParamsAs1DForOutWhenUnconnected=off
  wires:
  Demux3/14 -> Bus Creator3/14  "Vhcl Wheel RL Trq_WhlBearing"
  Demux3/13 -> Bus Creator3/13  "Vhcl Wheel RL Trq_T2W"
  Demux3/12 -> Bus Creator3/12  "Vhcl Wheel RL SideSlip"
  Demux3/11 -> Bus Creator3/11  "Vhcl Wheel RL LongSlip"
  Demux3/10 -> Bus Creator3/10  "Vhcl Wheel RL vBelt"
  Demux3/9 -> Bus Creator3/9  "Vhcl Wheel RL Fz"
  Demux3/8 -> Bus Creator3/8  "Vhcl Wheel RL Fy"
  Demux3/7 -> Bus Creator3/7  "Vhcl Wheel RL Fx"
  Demux3/6 -> Bus Creator3/6  "Vhcl Wheel RL r_zxy z"
  Demux3/5 -> Bus Creator3/5  "Vhcl Wheel RL r_zxy y"
  Demux3/4 -> Bus Creator3/4  "Vhcl Wheel RL r_zxy x"
  Demux3/3 -> Bus Creator3/3  "Vhcl Wheel RL t z"
  Demux3/2 -> Bus Creator3/2  "Vhcl Wheel RL t y"
  In1/1 -> Demux3/1
  Bus Creator3/1 -> Out1/1
  Demux3/1 -> Bus Creator3/1  "Vhcl Wheel RL t x"

== system generic_truck_src/TruckMaker/IPG Vehicle/CarAndTrailer/Trailer/CreateBus Vhcl.Wheel.RL2 ==
  In1 : Inport
  Bus Creator3 : BusCreator  Inputs=14
  Demux3 : Demux  Outputs=14
      settings: DisplayOption=none
  Out1 : Outport  VectorParamsAs1DForOutWhenUnconnected=off
  wires:
  Demux3/14 -> Bus Creator3/14  "Vhcl Wheel RL2 Trq_WhlBearing"
  Demux3/13 -> Bus Creator3/13  "Vhcl Wheel RL2 Trq_T2W"
  Demux3/12 -> Bus Creator3/12  "Vhcl Wheel RL2 SideSlip"
  Demux3/11 -> Bus Creator3/11  "Vhcl Wheel RL2 LongSlip"
  Demux3/10 -> Bus Creator3/10  "Vhcl Wheel RL2 vBelt"
  Demux3/9 -> Bus Creator3/9  "Vhcl Wheel RL2 Fz"
  Demux3/8 -> Bus Creator3/8  "Vhcl Wheel RL2 Fy"
  Demux3/7 -> Bus Creator3/7  "Vhcl Wheel RL2 Fx"
  Demux3/6 -> Bus Creator3/6  "Vhcl Wheel RL2 r_zxy z"
  Demux3/5 -> Bus Creator3/5  "Vhcl Wheel RL2 r_zxy y"
  Demux3/4 -> Bus Creator3/4  "Vhcl Wheel RL2 r_zxy x"
  Demux3/3 -> Bus Creator3/3  "Vhcl Wheel RL2 t z"
  Demux3/2 -> Bus Creator3/2  "Vhcl Wheel RL2 t y"
  In1/1 -> Demux3/1
  Bus Creator3/1 -> Out1/1
  Demux3/1 -> Bus Creator3/1  "Vhcl Wheel RL2 t x"

== system generic_truck_src/TruckMaker/IPG Vehicle/CarAndTrailer/Trailer/CreateBus Vhcl.Wheel.RL3 ==
  In1 : Inport
  Bus Creator3 : BusCreator  Inputs=14
  Demux3 : Demux  Outputs=14
      settings: DisplayOption=none
  Out1 : Outport  VectorParamsAs1DForOutWhenUnconnected=off
  wires:
  Demux3/1 -> Bus Creator3/1  "Vhcl Wheel RL3 t x"
  Bus Creator3/1 -> Out1/1
  In1/1 -> Demux3/1
  Demux3/2 -> Bus Creator3/2  "Vhcl Wheel RL3 t y"
  Demux3/3 -> Bus Creator3/3  "Vhcl Wheel RL3 t z"
  Demux3/4 -> Bus Creator3/4  "Vhcl Wheel RL3 r_zxy x"
  Demux3/5 -> Bus Creator3/5  "Vhcl Wheel RL3 r_zxy y"
  Demux3/6 -> Bus Creator3/6  "Vhcl Wheel RL3 r_zxy z"
  Demux3/7 -> Bus Creator3/7  "Vhcl Wheel RL3 Fx"
  Demux3/8 -> Bus Creator3/8  "Vhcl Wheel RL3 Fy"
  Demux3/9 -> Bus Creator3/9  "Vhcl Wheel RL3 Fz"
  Demux3/10 -> Bus Creator3/10  "Vhcl Wheel RL3 vBelt"
  Demux3/11 -> Bus Creator3/11  "Vhcl Wheel RL3 LongSlip"
  Demux3/12 -> Bus Creator3/12  "Vhcl Wheel RL3 SideSlip"
  Demux3/13 -> Bus Creator3/13  "Vhcl Wheel RL3 Trq_T2W"
  Demux3/14 -> Bus Creator3/14  "Vhcl Wheel RL3 Trq_WhlBearing"

== system generic_truck_src/TruckMaker/IPG Vehicle/CarAndTrailer/Trailer/CreateBus Vhcl.Wheel.RL4 ==
  In1 : Inport
  Bus Creator3 : BusCreator  Inputs=14
  Demux3 : Demux  Outputs=14
      settings: DisplayOption=none
  Out1 : Outport  VectorParamsAs1DForOutWhenUnconnected=off
  wires:
  Demux3/14 -> Bus Creator3/14  "Vhcl Wheel RL4 Trq_WhlBearing"
  Demux3/13 -> Bus Creator3/13  "Vhcl Wheel RL4 Trq_T2W"
  Demux3/12 -> Bus Creator3/12  "Vhcl Wheel RL4 SideSlip"
  Demux3/11 -> Bus Creator3/11  "Vhcl Wheel RL4 LongSlip"
  Demux3/10 -> Bus Creator3/10  "Vhcl Wheel RL4 vBelt"
  Demux3/9 -> Bus Creator3/9  "Vhcl Wheel RL4 Fz"
  Demux3/8 -> Bus Creator3/8  "Vhcl Wheel RL4 Fy"
  Demux3/7 -> Bus Creator3/7  "Vhcl Wheel RL4 Fx"
  Demux3/6 -> Bus Creator3/6  "Vhcl Wheel RL4 r_zxy z"
  Demux3/5 -> Bus Creator3/5  "Vhcl Wheel RL4 r_zxy y"
  Demux3/4 -> Bus Creator3/4  "Vhcl Wheel RL4 r_zxy x"
  Demux3/3 -> Bus Creator3/3  "Vhcl Wheel RL4 t z"
  Demux3/2 -> Bus Creator3/2  "Vhcl Wheel RL4 t y"
  In1/1 -> Demux3/1
  Bus Creator3/1 -> Out1/1
  Demux3/1 -> Bus Creator3/1  "Vhcl Wheel RL4 t x"

== system generic_truck_src/TruckMaker/IPG Vehicle/CarAndTrailer/Trailer/CreateBus Vhcl.Wheel.RR ==
  In1 : Inport
  Bus Creator3 : BusCreator  Inputs=14
  Demux3 : Demux  Outputs=14
      settings: DisplayOption=none
  Out1 : Outport  VectorParamsAs1DForOutWhenUnconnected=off
  wires:
  Demux3/14 -> Bus Creator3/14  "Vhcl Wheel RR Trq_WhlBearing"
  Demux3/13 -> Bus Creator3/13  "Vhcl Wheel RR Trq_T2W"
  Demux3/12 -> Bus Creator3/12  "Vhcl Wheel RR SideSlip"
  Demux3/11 -> Bus Creator3/11  "Vhcl Wheel RR LongSlip"
  Demux3/10 -> Bus Creator3/10  "Vhcl Wheel RR vBelt"
  Demux3/9 -> Bus Creator3/9  "Vhcl Wheel RR Fz"
  Demux3/8 -> Bus Creator3/8  "Vhcl Wheel RR Fy"
  Demux3/7 -> Bus Creator3/7  "Vhcl Wheel RR Fx"
  Demux3/6 -> Bus Creator3/6  "Vhcl Wheel RR r_zxy z"
  Demux3/5 -> Bus Creator3/5  "Vhcl Wheel RR r_zxy y"
  Demux3/4 -> Bus Creator3/4  "Vhcl Wheel RR r_zxy x"
  Demux3/3 -> Bus Creator3/3  "Vhcl Wheel RR t z"
  Demux3/2 -> Bus Creator3/2  "Vhcl Wheel RR t y"
  In1/1 -> Demux3/1
  Bus Creator3/1 -> Out1/1
  Demux3/1 -> Bus Creator3/1  "Vhcl Wheel RR t x"

== system generic_truck_src/TruckMaker/IPG Vehicle/CarAndTrailer/Trailer/CreateBus Vhcl.Wheel.RR2 ==
  In1 : Inport
  Bus Creator3 : BusCreator  Inputs=14
  Demux3 : Demux  Outputs=14
      settings: DisplayOption=none
  Out1 : Outport  VectorParamsAs1DForOutWhenUnconnected=off
  wires:
  Demux3/14 -> Bus Creator3/14  "Vhcl Wheel RR2 Trq_WhlBearing"
  Demux3/13 -> Bus Creator3/13  "Vhcl Wheel RR2 Trq_T2W"
  Demux3/12 -> Bus Creator3/12  "Vhcl Wheel RR2 SideSlip"
  Demux3/11 -> Bus Creator3/11  "Vhcl Wheel RR2 LongSlip"
  Demux3/10 -> Bus Creator3/10  "Vhcl Wheel RR2 vBelt"
  Demux3/9 -> Bus Creator3/9  "Vhcl Wheel RR2 Fz"
  Demux3/8 -> Bus Creator3/8  "Vhcl Wheel RR2 Fy"
  Demux3/7 -> Bus Creator3/7  "Vhcl Wheel RR2 Fx"
  Demux3/6 -> Bus Creator3/6  "Vhcl Wheel RR2 r_zxy z"
  Demux3/5 -> Bus Creator3/5  "Vhcl Wheel RR2 r_zxy y"
  Demux3/4 -> Bus Creator3/4  "Vhcl Wheel RR2 r_zxy x"
  Demux3/3 -> Bus Creator3/3  "Vhcl Wheel RR2 t z"
  Demux3/2 -> Bus Creator3/2  "Vhcl Wheel RR2 t y"
  In1/1 -> Demux3/1
  Bus Creator3/1 -> Out1/1
  Demux3/1 -> Bus Creator3/1  "Vhcl Wheel RR2 t x"

== system generic_truck_src/TruckMaker/IPG Vehicle/CarAndTrailer/Trailer/CreateBus Vhcl.Wheel.RR3 ==
  In1 : Inport
  Bus Creator3 : BusCreator  Inputs=14
  Demux3 : Demux  Outputs=14
      settings: DisplayOption=none
  Out1 : Outport  VectorParamsAs1DForOutWhenUnconnected=off
  wires:
  Demux3/1 -> Bus Creator3/1  "Vhcl Wheel RR3 t x"
  Bus Creator3/1 -> Out1/1
  In1/1 -> Demux3/1
  Demux3/2 -> Bus Creator3/2  "Vhcl Wheel RR3 t y"
  Demux3/3 -> Bus Creator3/3  "Vhcl Wheel RR3 t z"
  Demux3/4 -> Bus Creator3/4  "Vhcl Wheel RR3 r_zxy x"
  Demux3/5 -> Bus Creator3/5  "Vhcl Wheel RR3 r_zxy y"
  Demux3/6 -> Bus Creator3/6  "Vhcl Wheel RR3 r_zxy z"
  Demux3/7 -> Bus Creator3/7  "Vhcl Wheel RR3 Fx"
  Demux3/8 -> Bus Creator3/8  "Vhcl Wheel RR3 Fy"
  Demux3/9 -> Bus Creator3/9  "Vhcl Wheel RR3 Fz"
  Demux3/10 -> Bus Creator3/10  "Vhcl Wheel RR3 vBelt"
  Demux3/11 -> Bus Creator3/11  "Vhcl Wheel RR3 LongSlip"
  Demux3/12 -> Bus Creator3/12  "Vhcl Wheel RR3 SideSlip"
  Demux3/13 -> Bus Creator3/13  "Vhcl Wheel RR3 Trq_T2W"
  Demux3/14 -> Bus Creator3/14  "Vhcl Wheel RR3 Trq_WhlBearing"

== system generic_truck_src/TruckMaker/IPG Vehicle/CarAndTrailer/Trailer/CreateBus Vhcl.Wheel.RR4 ==
  In1 : Inport
  Bus Creator3 : BusCreator  Inputs=14
  Demux3 : Demux  Outputs=14
      settings: DisplayOption=none
  Out1 : Outport  VectorParamsAs1DForOutWhenUnconnected=off
  wires:
  Demux3/14 -> Bus Creator3/14  "Vhcl Wheel RR4 Trq_WhlBearing"
  Demux3/13 -> Bus Creator3/13  "Vhcl Wheel RR4 Trq_T2W"
  Demux3/12 -> Bus Creator3/12  "Vhcl Wheel RR4 SideSlip"
  Demux3/11 -> Bus Creator3/11  "Vhcl Wheel RR4 LongSlip"
  Demux3/10 -> Bus Creator3/10  "Vhcl Wheel RR4 vBelt"
  Demux3/9 -> Bus Creator3/9  "Vhcl Wheel RR4 Fz"
  Demux3/8 -> Bus Creator3/8  "Vhcl Wheel RR4 Fy"
  Demux3/7 -> Bus Creator3/7  "Vhcl Wheel RR4 Fx"
  Demux3/6 -> Bus Creator3/6  "Vhcl Wheel RR4 r_zxy z"
  Demux3/5 -> Bus Creator3/5  "Vhcl Wheel RR4 r_zxy y"
  Demux3/4 -> Bus Creator3/4  "Vhcl Wheel RR4 r_zxy x"
  Demux3/3 -> Bus Creator3/3  "Vhcl Wheel RR4 t z"
  Demux3/2 -> Bus Creator3/2  "Vhcl Wheel RR4 t y"
  In1/1 -> Demux3/1
  Bus Creator3/1 -> Out1/1
  Demux3/1 -> Bus Creator3/1  "Vhcl Wheel RR4 t x"

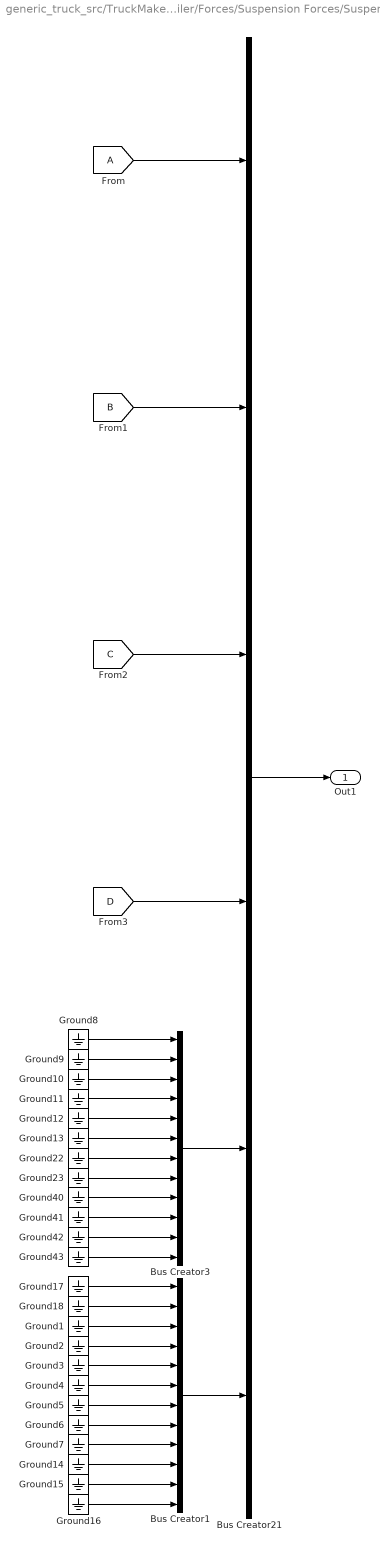
== system generic_truck_src/TruckMaker/IPG Vehicle/CarAndTrailer/Forces/Suspension Forces/Suspension External Forces Update ==
  Bus Creator1 : BusCreator  Inputs=12
  Bus Creator21 : BusCreator  Inputs=6
  Bus Creator3 : BusCreator  Inputs=12
  Ground{1..18,22..23,40..43} (24 alike) : Ground
  Out1 : Outport
  wires:
  Bus Creator21/1 -> Out1/1
  [C] -> Bus Creator21/3
  [B] -> Bus Creator21/2
  [A] -> Bus Creator21/1
  [D] -> Bus Creator21/4
  Ground22/1 -> Bus Creator3/7
  Ground12/1 -> Bus Creator3/5
  Ground10/1 -> Bus Creator3/3
  Ground8/1 -> Bus Creator3/1
  Ground40/1 -> Bus Creator3/9
  Ground23/1 -> Bus Creator3/8
  Ground41/1 -> Bus Creator3/10
  Ground9/1 -> Bus Creator3/2
  Bus Creator3/1 -> Bus Creator21/5
  Ground11/1 -> Bus Creator3/4
  Ground13/1 -> Bus Creator3/6
  Ground43/1 -> Bus Creator3/12
  Ground42/1 -> Bus Creator3/11
  Ground6/1 -> Bus Creator1/8
  Ground7/1 -> Bus Creator1/9
  Ground3/1 -> Bus Creator1/5
  Ground15/1 -> Bus Creator1/11
  Ground14/1 -> Bus Creator1/10
  Ground4/1 -> Bus Creator1/6
  Ground2/1 -> Bus Creator1/4
  Ground16/1 -> Bus Creator1/12
  Ground18/1 -> Bus Creator1/2
  Bus Creator1/1 -> Bus Creator21/6
  Ground5/1 -> Bus Creator1/7
  Ground17/1 -> Bus Creator1/1
  Ground1/1 -> Bus Creator1/3
